simulink model "satuSystm"  (R2024a)
settings: Solver=VariableStepAuto  StartTime=0.0  StopTime=5  RelTol=1e-3
settings Model: Creator=farza  LastModifiedBy=farza

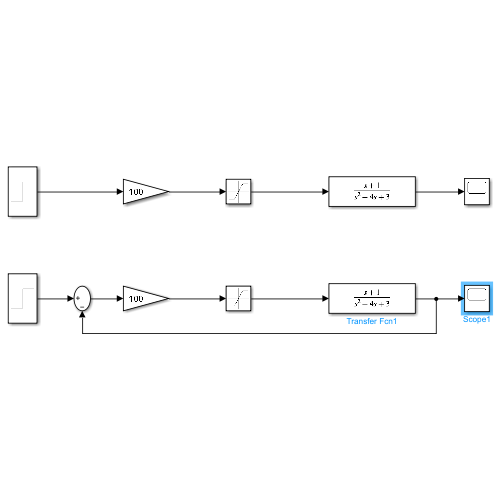
[thumbnail: Simulink's stored preview of the top-level diagram]
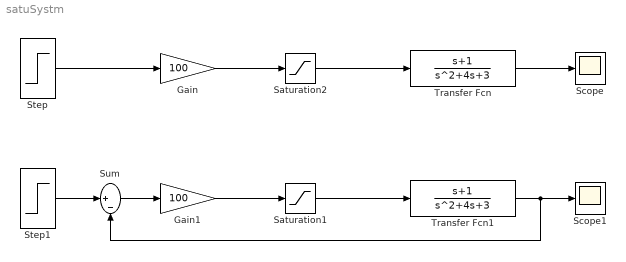
== system satuSystm ==
  Gain : Gain  Gain=100
  Gain1 : Gain  Gain=100
  Saturation1 : Saturate  UpperLimit=5  LowerLimit=-5
  Saturation2 : Saturate  UpperLimit=5  LowerLimit=-5
  Scope : Scope
  Scope1 : Scope
  Step : Step  SampleTime=0
  Step1 : Step  SampleTime=0
  Sum : Sum  Inputs=|+-
  Transfer Fcn : TransferFcn  Numerator=[1 1]  Denominator=[1 4 3]
  Transfer Fcn1 : TransferFcn  Numerator=[1 1]  Denominator=[1 4 3]
  wires:
  Step/1 -> Gain/1
  Gain/1 -> Saturation2/1
  Saturation2/1 -> Transfer Fcn/1
  Transfer Fcn/1 -> Scope/1
  Saturation1/1 -> Transfer Fcn1/1
  Gain1/1 -> Saturation1/1
  Step1/1 -> Sum/1
  Sum/1 -> Gain1/1
  Transfer Fcn1/1 -> Sum/2, Scope1/1
